simulink model "test_model"  (R2023a)
settings: Solver=VariableStepAuto  StartTime=0.0  StopTime=138550  RelTol=1e-3
values from neighbouring files (symbols this model uses):
  T1 = 10    [L_delta_model.m]
  Ti = 10    [L_delta_model.m]
  V = 10    [L_delta_model.m]
libraries: opclib x1
settings Model: Creator=Yuganshu Wadhwa  LastModifiedBy=Yuganshu Wadhwa
settings DebuggingCC: UnconnectedInputMsg=warning  UnconnectedOutputMsg=warning  UnconnectedLineMsg=warning
settings ModelReferenceCC: EnableRefExpFcnMdlSchedulingChecks=on
settings RTWCC: DLArmComputeVersion=19.05

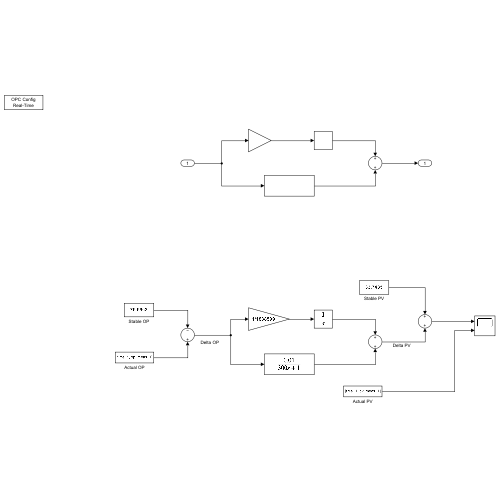
[thumbnail: Simulink's stored preview of the top-level diagram]
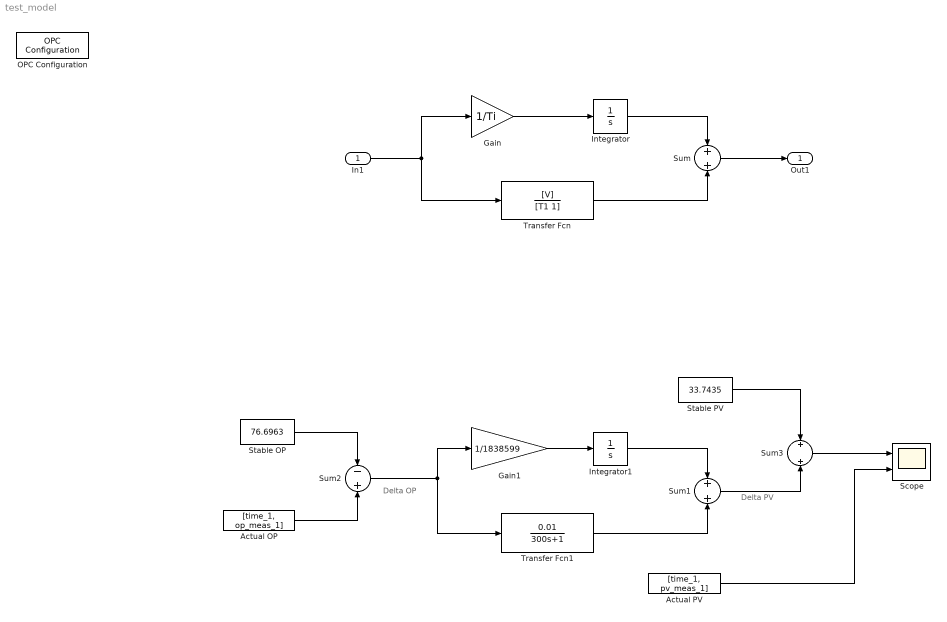
== system test_model ==
  note: Delta OP
  note: Delta PV
  In1 : Inport
  Actual OP : FromWorkspace  VariableName=[time_1, op_meas_1]
  Actual PV : FromWorkspace  VariableName=[time_1, pv_meas_1]
  Gain : Gain  Gain=1/Ti
  Gain1 : Gain  Gain=1/1838599
  Integrator : Integrator
  Integrator1 : Integrator
  OPC Configuration : opclib/OPC Configuration  errMissingItems=Error  errReadWrite=Warn  errShutdown=Error  errRTViolation=Warn  rtEnable=on  speedup=1  showLatency=off  beingUsed=on
  Scope : Scope  NumInputPorts=2
  Stable OP : Constant  Value=76.6963
  Stable PV : Constant  Value=33.7435
  Sum : Sum  Inputs=+|+
  Sum1 : Sum  Inputs=+|+
  Sum2 : Sum  Inputs=-|+
  Sum3 : Sum  Inputs=+|||+
  Transfer Fcn : TransferFcn  Numerator=[V]  Denominator=[T1 1]
  Transfer Fcn1 : TransferFcn  Numerator=[0.01]  Denominator=[300 1]
  Out1 : Outport
  wires:
  Gain/1 -> Integrator/1
  Integrator/1 -> Sum/1
  Transfer Fcn/1 -> Sum/2
  Sum/1 -> Out1/1
  In1/1 -> Transfer Fcn/1, Gain/1
  Gain1/1 -> Integrator1/1
  Integrator1/1 -> Sum1/1
  Transfer Fcn1/1 -> Sum1/2
  Actual PV/1 -> Scope/2
  Actual OP/1 -> Sum2/2
  Stable OP/1 -> Sum2/1
  Sum2/1 -> Transfer Fcn1/1, Gain1/1
  Sum1/1 -> Sum3/2
  Stable PV/1 -> Sum3/1
  Sum3/1 -> Scope/1
